simulink model "IonSatSimulation_ne_marche_pas_version_robin-lx-tavant.lab-lpp.local"  (R2019a)
settings: Solver=ode3  StartTime=0.0  StopTime=10000  FixedStep=.25  MaxStep=30  MinStep=.1  RelTol=1e-3
PreLoadFcn:
  | load('.\Data\SatConstants.mat')
model workspace (MAT data in the model file):
  repartition_matrix = Simulink.Parameter
  repartition_matrix.DataType = 'auto'
  repartition_matrix.Dimensions = [0 0]
  wheel_number = Simulink.Parameter
  wheel_number.Value = 3
  wheel_number.DataType = 'auto'
  wheel_number.Dimensions = [1 1]
undefined symbols (not defined in the file): Angle, Axis, deg, DiscIntNeverNeededParam, IAU, km, m, mu_Earth, rad, s, sat, X, Y, Z
libraries: aerolibutil x29, sm_lib x19, nesl_utility x16, aerolibconvert2 x13, vrlib x10, simulink x9, dspmathops x8, sharedtransform x7, sharedutil x5, aerolibgravity2 x4, sharedTrackingLibrary x2, aerolibcelestial x2
(part 1 of 3)
settings Model: SnapshotBufferSize=100  OrderedModelArguments=off  Creator=robin  LastModifiedBy=robin
settings SolverCC: InitialStep=.5  MaxConsecutiveMinStep=2
settings DataIOCC: SaveFormat=StructureWithTime  SaveOutput=off  SignalLogging=off  DSMLogging=off  SaveTime=off
settings OptimizationCC: DefaultParameterBehavior=Inlined  UseDivisionForNetSlopeComputation=on  GainParamInheritBuiltInType=on  UseFloatMulNetSlope=on  InlineInvariantSignals=on  PassReuseOutputArgsAs=Individual arguments  ZeroExternalMemoryAtStartup=off  ZeroInternalMemoryAtStartup=off  NoFixptDivByZeroProtection=on  EfficientFloat2IntCast=on  LifeSpan=1  OptimizeBlockOrder=speed  DifferentSizesBufferReuse=on
settings DebuggingCC: ParameterTunabilityLossMsg=error
settings HardwareCC: ProdBitPerInt=16  ProdBitPerPointer=8  ProdBitPerSizeT=24  ProdBitPerPtrDiffT=24  ProdLargestAtomicFloat=None  ProdWordSize=8  ProdLongLongMode=on  ProdHWDeviceType=Microchip->PIC18
settings SFSimCC: MATLABDynamicMemAlloc=off
settings RTWCC: SystemTargetFile=ert.tlc  TemplateMakefile=ert_default_tmf  GenerateReport=on  IncludeHyperlinkInReport=on  LaunchReport=on  GenerateTraceInfo=on  GenerateTraceReport=on  GenerateTraceReportSl=on  GenerateTraceReportSf=on  GenerateTraceReportEml=on  GenerateCodeMetricsReport=on
settings CodeAppCC: ForceParamTrailComments=on  IgnoreCustomStorageClasses=off  OperatorAnnotations=on  SimulinkDataObjDesc=on  SFDataObjDesc=on  CustomSymbolStrGlobalVar=rt$N$M  CustomSymbolStrType=$N$M  CustomSymbolStrFcn=$N$M$F  CustomSymbolStrMacro=$N$M  InsertBlockDesc=on
settings ERTTargetCC: TargetLangStandard=C99 (ISO)  GenerateSampleERTMain=on  IncludeMdlTerminateFcn=off  CombineSignalStateStructs=on  SupportAbsoluteTime=off  SupportComplex=off  SupportContinuousTime=on  SupportNonInlinedSFcns=on  InlinedParameterPlacement=NonHierarchical  ERTCustomFileTemplate=example_file_process.tlc  ERTFilePackagingFormat=CompactWithDataFile

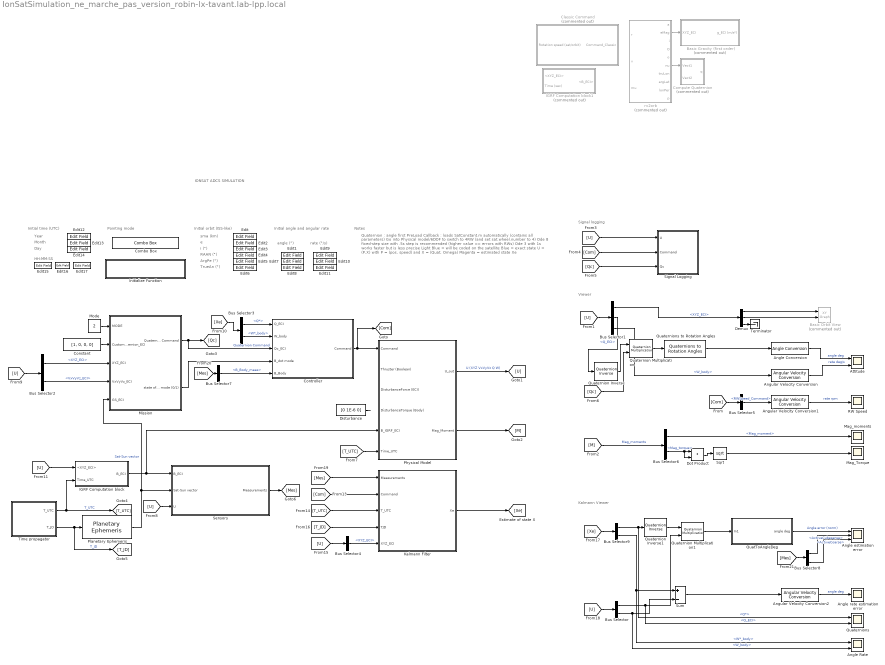
== system IonSatSimulation_ne_marche_pas_version_robin-lx-tavant.lab-lpp.local ==
  note: Kalmann Viewer
  note: IONSAT ADCS SIMULATION
  note: Viewer
  note: Pointing mode
  note: Initial orbit (ISS-like)
  note: sma (km)
  note: e
  note: i (°)
  note: RAAN (°)
  note: ArgPe (°)
  note: TrueAn (°)
  note: Initial angle and angular rate
  note: angle (°)
  note: rate (°/s)
  note: Notes
  note: Quaternion : angle first
      | PreLoad Callback : loads SatConstant.m automatically (contains all parameters)
      | Go into Physical model/6DOF to switch to 4RW (and set sat.wheel.number to 4)
      | Ode 8 fixed-step size with .5s step is recommended (higher value => errors with RWs)
      | Ode 3 with 1s works faster but is less precise
      | Light Blue = will be coded on the satellite
      | Blue = exact state U = (P,X) with P = (pos, speed) and X = (Quat, Omega)
      | Magenta = estimated state Xe
  note: Signal logging
  note: Month
  note: Year
  note: Day
  note: Initial time (UTC)
  note: HH:MM:SS
  Angle Conversion : aerolibconvert2/Angle Conversion  IU=rad  OU=deg
  Angle Rate : Scope  NumInputPorts=2
  Angle estimation error : Scope  NumInputPorts=3
  Angle rate estimation error : Scope
  Angular Velocity Conversion : aerolibconvert2/Angular Velocity Conversion  IU=rad/s  OU=deg/s
      settings: SourceProductName=Aerospace Blockset
  Angular Velocity Conversion1 : aerolibconvert2/Angular Velocity Conversion  IU=rad/s  OU=rpm
      settings: SourceProductName=Aerospace Blockset
  Angular Velocity Conversion2 : aerolibconvert2/Angular Velocity Conversion  IU=rad/s  OU=deg/s
      settings: SourceProductName=Aerospace Blockset
  Attitude : Scope  NumInputPorts=2
  Basic Gravity (first order) : Subsystem  Commented=on
  Basic Orbit View : simulink/Sinks/XY Graph  Commented=on  xmin=-10000000  xmax=10000000  ymin=-10000000  ymax=10000000  st=-1
  Bus Selector : BusSelector  OutputSignals=Q_ECI,W_body
  Bus Selector1 : BusSelector  OutputSignals=XYZ_ECI,Q_ECI,W_body
  Bus Selector2 : BusSelector  OutputSignals=XYZ_ECI,VxVyVz_ECI
  Bus Selector3 : BusSelector  OutputSignals=Q*,W*_body
  Bus Selector4 : BusSelector  OutputSignals=XYZ_ECI
  Bus Selector5 : BusSelector  OutputSignals=RWSpeed_Command
  Bus Selector6 : BusSelector  OutputSignals=Mag_moment,Mag_torque
  Bus Selector7 : BusSelector  OutputSignals=B_Body_meas
  Bus Selector8 : BusSelector  OutputSignals=ActiveCubesense,ActiveCoarse
  Bus Selector9 : BusSelector  OutputSignals=Q*,W*_body
  Classic Command : Subsystem  Commented=on
  Combo Box : ComboBox  LabelPosition=Hide  SelectedLabel=Sun Aero
      settings: Values={{'Nadir', 'Retrograde', 'Drag', 'Sun', 'Sun Aero', 'B-dot', 'Custom Quaternion'}, [1 5 4 3 2 6 7]}
  Compute Quaternion : Subsystem  Commented=on
  Constant : Constant  Value=[1, 0, 0, 0]
  Controller : Subsystem  TreatAsAtomicUnit=on
  Demux : Demux  Outputs=3
  Disturbance : Constant  Value=[0 1E-6 0]
  Dot Product : DotProduct  InputSameDT=on  OutDataTypeStr=Inherit: Inherit via internal rule
  Edit{,1..17} (18 alike) : EditField  LabelPosition=Hide  ShowInitialText=on  Alignment=Center
  IGRF Computation block : Subsystem
  IGRF Computation block1 : Subsystem  Commented=on
  Initialize Function : Subsystem  TreatAsAtomicUnit=on
  Kalmann Filter : Subsystem  TreatAsAtomicUnit=on  SystemSampleTime=1
  Mag_Torque : Scope
  Mag_moments : Scope
  Mission : Subsystem  TreatAsAtomicUnit=on  SystemSampleTime=1
  Mode : Constant  Value=2  OutDataTypeStr=int8
  Physical Model : Subsystem
      settings: MinAlgLoopOccurrences=on
  Planetary Ephemeris : aerolibcelestial/Planetary Ephemeris  kmflag=km,km/s  epochflag=Julian date  de=DE405  nCenter=Earth  nTarget=Sun  errorflag=Error  velflag=off
      settings: SourceProductName=Aerospace Blockset  SourceProductBaseCode=AE
  QuatToAngleDeg : Subsystem
  Quaternion Inverse : aerolibutil/Quaternion Inverse
      settings: SourceProductName=Aerospace Blockset
  Quaternion Inverse1 : aerolibutil/Quaternion Inverse
      settings: SourceProductName=Aerospace Blockset
  Quaternion Multiplication : aerolibutil/Quaternion Multiplication
  Quaternion Multiplication1 : aerolibutil/Quaternion Multiplication
  Quaternions : Scope  NumInputPorts=2
  Quaternions to Rotation Angles : sharedtransform/Quaternions to Rotation Angles  rotationOrder=ZYX  aMode=aMode
      settings: SourceProductBaseCode=AE
  RW Speed : Scope
  Sensors : Subsystem
  Signal Logging : Subsystem
  Sqrt : Sqrt  SaturateOnIntegerOverflow=on
  Sum : Sum  Inputs=+-
  Terminator : Terminator
  Time propagator : Subsystem
  rv2orb : MATLAB Function  Commented=on  TreatAsAtomicUnit=on
  wires:
  Mission/1(Quaternion Command) -> [Qc], Controller/3(Qc_ECI)  "Quaternion Command"
  Mode/1 -> Mission/1(MODE)
  Bus Selector2/2 -> Mission/4(VxVyVz_ECI)  "<VxVyVz_ECI>"
  Physical Model/1(U_out) -> [U]  "U (XYZ VxVyVz Q W)"
  Controller/1(Command) -> [Com], Physical Model/1(Command)
  Angle Conversion/1 -> Attitude/1  "angle deg"
  Demux/3 -> Terminator/1
  Demux/2 -> Basic Orbit View/2
  Angular Velocity Conversion/1 -> Attitude/2  "rate deg/s"
  Bus Selector1/1 -> Demux/1  "<XYZ_ECI>"
  Quaternion Multiplication/1 -> Quaternions to Rotation Angles/1
  Demux/1 -> Basic Orbit View/1
  Bus Selector1/3 -> Angular Velocity Conversion/1  "<W_body>"
  Quaternions to Rotation Angles/1 -> Angle Conversion/1
  Angular Velocity Conversion1/1 -> RW Speed/1  "rate rpm"
  [Com] -> Bus Selector5/1
  [U] -> Bus Selector1/1
  rv2orb/2(eMag) -> Basic Gravity (first order)/1(XYZ_ECI)
  Bus Selector2/1 -> Mission/3(XYZ_ECI)  "<XYZ_ECI>"
  rv2orb/6(nu) -> Compute Quaternion/1(Vect1)
  Bus Selector3/1 -> Controller/1(Q_ECI)  "<Q*>"
  Bus Selector3/2 -> Controller/2(W_body)  "<W*_body>"
  Planetary Ephemeris/1 -> Mission/5(GS_ECI), Sensors/2(Sat-Sun vector)  "Sat-Sun vector"
  [U] -> Signal Logging/1(U)
  [Com] -> Signal Logging/2(Command)
  [Qc] -> Signal Logging/3(Qc)
  [Qc] -> Quaternion Multiplication/2
  Quaternion Inverse/1 -> Quaternion Multiplication/1
  Bus Selector1/2 -> Quaternion Inverse/1  "<Q_ECI>"
  Physical Model/2(Mag_Moment) -> [M]
  [M] -> Bus Selector6/1  "Mag_moments"
  Time propagator/1(T_UTC) -> [T_UTC], IGRF Computation block/2("Time_UTC ")  "T_UTC"
  Time propagator/2(T_JD) -> [T_JD], Planetary Ephemeris/1  "T_JD"
  Disturbance/1 -> ?
  Mission/2(state of B-dot mode (0/1)) -> Controller/4(B_dot mode)
  IGRF Computation block/1(B_ECI) -> Physical Model/5(B_IGRF_ECI), Sensors/1(B_ECI)
  Constant/1 -> Mission/2(Custom Quaternion_ECI)
  [T_UTC] -> Physical Model/6(Time_UTC)
  [U] -> Bus Selector2/1
  [Xe] -> Bus Selector3/1
  [U] -> IGRF Computation block/1(<XYZ_ECI>)
  Kalmann Filter/1(Xe) -> [Xe]
  [Com] -> Kalmann Filter/2(Command)
  [T_UTC] -> Kalmann Filter/3(T_UTC)
  [U] -> Bus Selector4/1
  Bus Selector4/1 -> Kalmann Filter/5(XYZ_ECI)  "<XYZ_ECI>"
  [T_JD] -> Kalmann Filter/4(TJD)
  [Xe] -> Bus Selector9/1
  [U] -> Bus Selector/1
  Bus Selector9/2 -> Angle Rate/1, Sum/1  "<W*_body>"
  Bus Selector/2 -> Angle Rate/2, Sum/2  "<W_body>"
  Sum/1 -> Angular Velocity Conversion2/1
  Bus Selector9/1 -> Quaternions/1, Quaternion Inverse1/1  "<Q*>"
  Quaternion Inverse1/1 -> Quaternion Multiplication1/1
  Bus Selector/1 -> Quaternions/2, Quaternion Multiplication1/2  "<Q_ECI>"
  Angular Velocity Conversion2/1 -> Angle rate estimation error/1  "angle deg"
  Bus Selector5/1 -> Angular Velocity Conversion1/1  "<RWSpeed_Command>"
  Bus Selector6/1 -> Mag_moments/1  "<Mag_moment>"
  Bus Selector6/2 -> Dot Product/2, Dot Product/1  "<Mag_torque>"
  Dot Product/1 -> Sqrt/1
  Sqrt/1 -> Mag_Torque/1
  Bus Selector7/1 -> Controller/5(B_Body)  "<B_Body_meas>"
  [U] -> Sensors/3(U)
  Sensors/1(Measurements) -> [Mes]
  [Mes] -> Kalmann Filter/1(Measurements)
  [Mes] -> Bus Selector7/1
  [Mes] -> Bus Selector8/1
  Bus Selector8/1 -> Angle estimation error/2  "<ActiveCubesense>"
  Bus Selector8/2 -> Angle estimation error/3  "<ActiveCoarse>"
  Quaternion Multiplication1/1 -> QuatToAngleDeg/1(In1)
  QuatToAngleDeg/1(angle deg) -> Angle estimation error/1  "Angle error (norm)"

== system IonSatSimulation_ne_marche_pas_version_robin-lx-tavant.lab-lpp.local/Basic Gravity (first order) ==
  XYZ_ECI : Inport
  Constant : Constant  Value=-mu_Earth
  Constant3 : Constant  Value=3/2
  Divide : Product  Inputs=*/
  Norm : Subsystem
  Product : Product
  Square3 : Math  Operator=pow  SaturateOnIntegerOverflow=on
  g_ECI (m/s²) : Outport  VectorParamsAs1DForOutWhenUnconnected=on
  wires:
  Constant/1 -> Divide/1
  Divide/1 -> Product/2
  Product/1 -> g_ECI (m/s²)/1
  XYZ_ECI/1 -> Norm/1(u), Product/1
  Square3/1 -> Divide/2  "r**3"
  Constant3/1 -> Square3/2
  Norm/1(r**2) -> Square3/1

== system IonSatSimulation_ne_marche_pas_version_robin-lx-tavant.lab-lpp.local/Classic Command ==
  Rotation speed (sat/orbit) : Inport
  Gain : Gain  Gain=- sat.PID.k_mag_classic
  Command_Classic : Outport
  wires:
  Rotation speed (sat/orbit)/1 -> Gain/1
  Gain/1 -> Command_Classic/1

== system IonSatSimulation_ne_marche_pas_version_robin-lx-tavant.lab-lpp.local/Compute Quaternion ==
  Vect1 : Inport
  Vect2 : Inport  Port=2
  Constant : Constant
  Cross Product : vrlib/Utilities/Cross Product
      settings: SourceProductName=Simulink
  Dot Product : DotProduct  InputSameDT=on  OutDataTypeStr=Inherit: Inherit via internal rule
  Mux : Mux  Inputs=2
  Normalization : dspmathops/Normalization  NormType=2-norm  Bias=1e-10  NormOver=Each column  Dimension=1  roundingMode=Floor  overflowMode=off  accumDataTypeStr=Inherit: Same as product output  accumLastDataTypeStr=Inherit: Same as product output  outputDataTypeStr=Inherit: Same as product output  outputMin=[]  outputMax=[]  outputLastDataTypeStr=Inherit: Same as product output
      settings: SourceProductName=DSP System Toolbox
  Normalization1 : dspmathops/Normalization  NormType=2-norm  Bias=1e-10  NormOver=Each column  Dimension=1  roundingMode=Floor  overflowMode=off  accumDataTypeStr=Inherit: Same as product output  accumLastDataTypeStr=Inherit: Same as product output  outputDataTypeStr=Inherit: Same as product output  outputMin=[]  outputMax=[]  outputLastDataTypeStr=Inherit: Same as product output
      settings: SourceProductName=DSP System Toolbox
  Quaternion Normalize : sharedutil/Quaternion Normalize  aMode=aMode
      settings: SourceProductName=Aerospace Blockset  SourceProductBaseCode=AE
  Sum : Sum  Inputs=|++
  q : Outport  PortDimensions=4
  wires:
  Vect1/1 -> Normalization/1
  Normalization/1 -> Cross Product/1, Dot Product/1
  Vect2/1 -> Normalization1/1
  Normalization1/1 -> Dot Product/2, Cross Product/2
  Cross Product/1 -> Mux/2
  Dot Product/1 -> Sum/1
  Sum/1 -> Mux/1
  Constant/1 -> Sum/2
  Mux/1 -> Quaternion Normalize/1
  Quaternion Normalize/1 -> q/1

== system IonSatSimulation_ne_marche_pas_version_robin-lx-tavant.lab-lpp.local/Controller ==
  note: Choix d'un contrôleur PID : plus simple et robuste qu'un LQR/SliddingSurface ou autre
  note: Runs as fast as possible
  note: Runs at 1Hz
  Q_ECI : Inport
  W_body : Inport  Port=2
  Qc_ECI : Inport  Port=3
  B_dot mode : Inport  Port=4
  B_Body : Inport  Port=5
  B-dot choice1 : Subsystem
  B-dot choice2 : Subsystem
  B-dot command : Subsystem  TreatAsAtomicUnit=on
  Bus Creator : BusCreator  Inputs=2
  Ground2 : Ground  Commented=on
  PID (nominal command) : Subsystem  TreatAsAtomicUnit=on  SystemSampleTime=1
  RW4 : Subsystem  Commented=on
  Command : Outport
  wires:
  Ground2/1 -> RW4/1(Mc (scalar))
  B_Body/1 -> B-dot command/1(B), PID (nominal command)/4(B_IGRF_Body)
  B-dot choice2/1(output command) -> Bus Creator/2  "Magnetotorquer_Command"
  B-dot choice1/1(output command) -> Bus Creator/1  "RWSpeed_Command"
  B-dot command/2(Wheel command (0)) -> B-dot choice1/2(Command (B-dot))
  B-dot command/1(Magnetic moment (B-dot)) -> B-dot choice2/2(Command (B-dot))
  B_dot mode/1 -> B-dot choice2/3(B_dot mode (0/1)), B-dot choice1/3(B_dot mode (0/1))
  Q_ECI/1 -> PID (nominal command)/1(Q_ECI)
  Qc_ECI/1 -> PID (nominal command)/2(Qc_ECI)
  W_body/1 -> PID (nominal command)/3(W_Body)
  PID (nominal command)/1(RW Command) -> B-dot choice1/1(" command (normal)")
  PID (nominal command)/2(Mag Command) -> B-dot choice2/1(" command (normal)")
  Bus Creator/1 -> Command/1

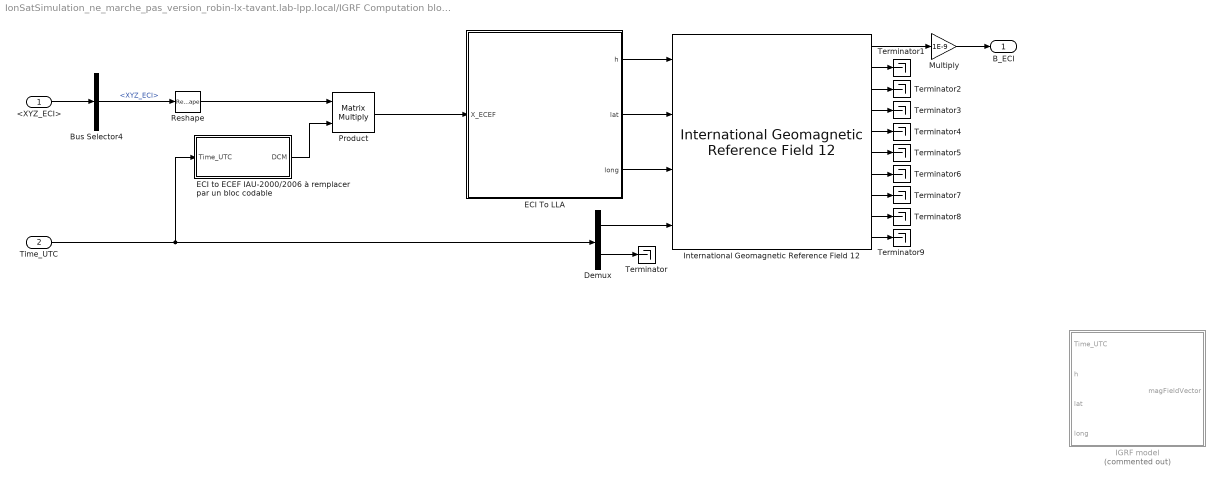
== system IonSatSimulation_ne_marche_pas_version_robin-lx-tavant.lab-lpp.local/IGRF Computation block ==
  <XYZ_ECI> : Inport
  "Time_UTC " : Inport  Port=2
  Bus Selector4 : BusSelector  OutputSignals=XYZ_ECI
  Demux : Demux  Outputs=2
  ECI To LLA : MATLAB Function  TreatAsAtomicUnit=on
  ECI to ECEF IAU-2000/2006 à remplacer par un bloc codable : MATLAB Function  TreatAsAtomicUnit=on
  IGRF model : MATLAB Function  Commented=on  TreatAsAtomicUnit=on
  International Geomagnetic Reference Field 12 : aerolibgravity2/International Geomagnetic Reference Field 12  units=Metric (MKS)  time_in=on  month=January  day=1  year=2020  action=None  sv_out=on
      settings: SourceProductName=Aerospace Blockset  SourceProductBaseCode=AE
  Multiply : Gain  Gain=1E-9
  Product : Product  Multiplication=Matrix(*)
  Reshape : Reshape  OutputDimensionality=Row vector (2-D)
  Terminator{,1..9} (10 alike) : Terminator
  B_ECI : Outport
  wires:
  ECI To LLA/3(long) -> International Geomagnetic Reference Field 12/3
  ECI To LLA/2(lat) -> International Geomagnetic Reference Field 12/2
  ECI To LLA/1(h) -> International Geomagnetic Reference Field 12/1
  International Geomagnetic Reference Field 12/1 -> Multiply/1
  Demux/1 -> International Geomagnetic Reference Field 12/4
  Demux/2 -> Terminator/1
  International Geomagnetic Reference Field 12/2 -> Terminator1/1
  International Geomagnetic Reference Field 12/3 -> Terminator2/1
  International Geomagnetic Reference Field 12/4 -> Terminator3/1
  International Geomagnetic Reference Field 12/5 -> Terminator4/1
  International Geomagnetic Reference Field 12/6 -> Terminator5/1
  International Geomagnetic Reference Field 12/7 -> Terminator6/1
  International Geomagnetic Reference Field 12/8 -> Terminator7/1
  International Geomagnetic Reference Field 12/9 -> Terminator8/1
  International Geomagnetic Reference Field 12/10 -> Terminator9/1
  Multiply/1 -> B_ECI/1
  ECI to ECEF IAU-2000/2006 à remplacer par un bloc codable/1(DCM) -> Product/2
  "Time_UTC "/1 -> Demux/1, ECI to ECEF IAU-2000/2006 à remplacer par un bloc codable/1(Time_UTC)
  <XYZ_ECI>/1 -> Bus Selector4/1
  Reshape/1 -> Product/1
  Product/1 -> ECI To LLA/1(X_ECEF)
  Bus Selector4/1 -> Reshape/1  "<XYZ_ECI>"

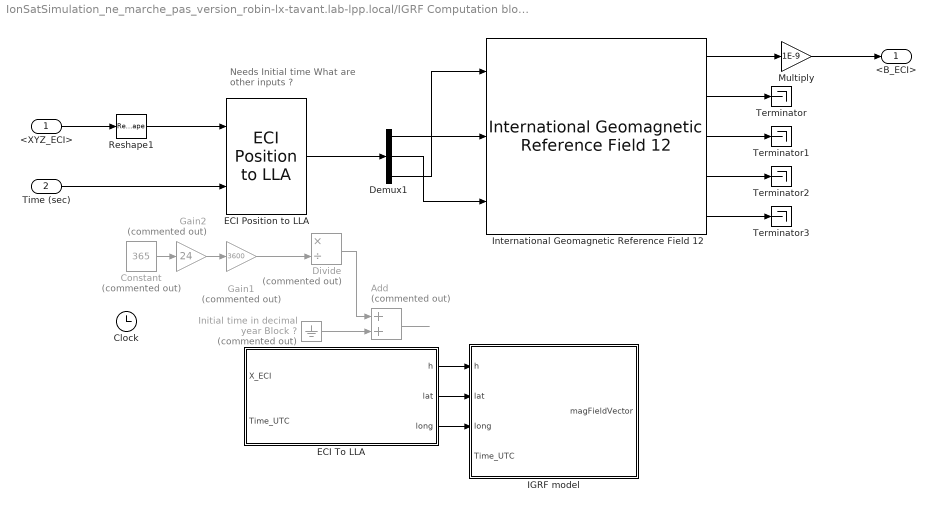
== system IonSatSimulation_ne_marche_pas_version_robin-lx-tavant.lab-lpp.local/IGRF Computation block1 ==
  note: Needs Initial time
      | What are other inputs ?
  <XYZ_ECI> : Inport
  Time (sec) : Inport  Port=2
  Add : Sum  Commented=on
  Clock : Clock
  Constant : Constant  Commented=on  Value=365
  Demux1 : Demux  Outputs=3
  Divide : Product  Commented=on  Inputs=*/
  ECI Position to LLA : aerolibtransform2/ECI Position to LLA  red=IAU-2000/2006  year=2020  month=January  day=1  hour=0  min=0  sec=0  deltaT=Sec  errorflag=Error  extraparamflag=off  eunits=Metric (MKS)  earthmodel=WGS84  flat=1/298.257223563  eqradius=6378137
      settings: AttributesFormatString=%<red>  SourceProductName=Aerospace Blockset  SourceProductBaseCode=AE
  ECI To LLA : MATLAB Function  TreatAsAtomicUnit=on
  Gain1 : Gain  Commented=on  Gain=3600
  Gain2 : Gain  Commented=on  Gain=24
  IGRF model : MATLAB Function  TreatAsAtomicUnit=on
  Initial time in decimal year Block ? : Ground  Commented=on
  International Geomagnetic Reference Field 12 : aerolibgravity2/International Geomagnetic Reference Field 12  units=Metric (MKS)  time_in=off  month=January  day=1  year=2020  action=None  sv_out=off
      settings: SourceProductName=Aerospace Blockset  SourceProductBaseCode=AE
  Multiply : Gain  Gain=1E-9
  Reshape1 : Reshape  OutputDimensionality=Column vector (2-D)
  Terminator{,1..3} (4 alike) : Terminator
  <B_ECI> : Outport
  wires:
  International Geomagnetic Reference Field 12/1 -> Multiply/1
  Demux1/2 -> International Geomagnetic Reference Field 12/3
  Time (sec)/1 -> ECI Position to LLA/2
  ECI Position to LLA/1 -> Demux1/1
  <XYZ_ECI>/1 -> Reshape1/1
  Gain2/1 -> Gain1/1
  Constant/1 -> Gain2/1
  Gain1/1 -> Divide/2
  Add/1 -> ?
  Divide/1 -> Add/1
  Initial time in decimal year Block ?/1 -> Add/2
  Reshape1/1 -> ECI Position to LLA/1
  International Geomagnetic Reference Field 12/3 -> Terminator1/1
  International Geomagnetic Reference Field 12/2 -> Terminator/1
  International Geomagnetic Reference Field 12/4 -> Terminator2/1
  International Geomagnetic Reference Field 12/5 -> Terminator3/1
  Demux1/1 -> International Geomagnetic Reference Field 12/2
  Demux1/3 -> International Geomagnetic Reference Field 12/1
  Multiply/1 -> <B_ECI>/1
  ECI To LLA/3(long) -> IGRF model/3(long)
  ECI To LLA/2(lat) -> IGRF model/2(lat)
  ECI To LLA/1(h) -> IGRF model/1(h)

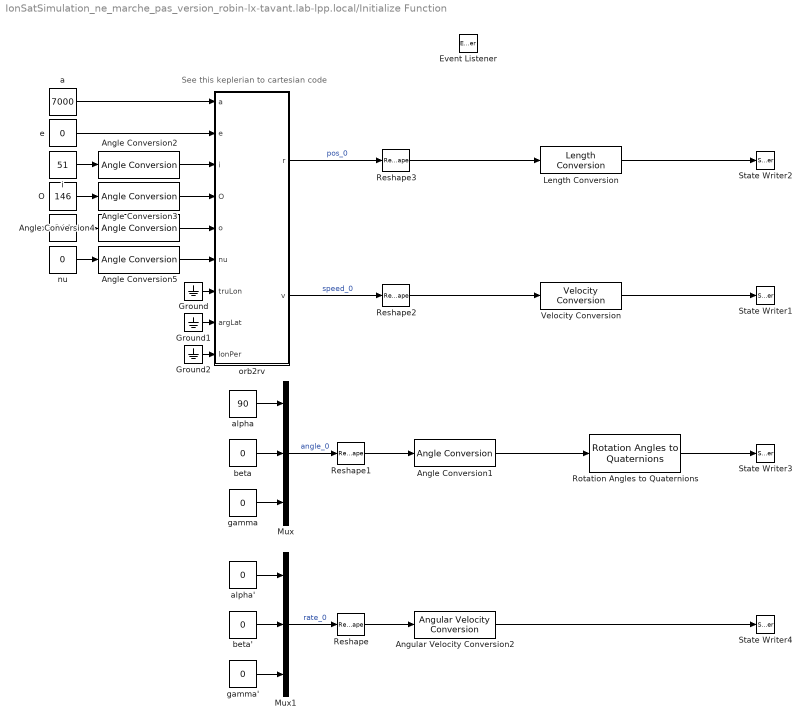
== system IonSatSimulation_ne_marche_pas_version_robin-lx-tavant.lab-lpp.local/Initialize Function ==
  note: See this keplerian to cartesian code
  Angle Conversion{1..5} (5 alike) : aerolibconvert2/Angle Conversion  IU=deg  OU=rad
  Angular Velocity Conversion2 : aerolibconvert2/Angular Velocity Conversion  IU=deg/s  OU=rad/s
      settings: SourceProductName=Aerospace Blockset
  Event Listener : EventListener  DisableCoverage=on  EventName=reset
  Ground : Ground
  Ground1 : Ground
  Ground2 : Ground
  Length Conversion : aerolibconvert2/Length Conversion  IU=km  OU=m
  Mux : Mux  Inputs=3
  Mux1 : Mux  Inputs=3
  O : Constant  Value=146
  Reshape{,1..3} (4 alike) : Reshape  OutputDimensionality=Column vector (2-D)
  Rotation Angles to Quaternions : sharedtransform/Rotation Angles to Quaternions  rotationOrder=ZYX  aMode=aMode
      settings: SourceProductName=Aerospace Blockset  SourceProductBaseCode=AE
  State Writer1 : StateWriter  StateOwnerBlock=../../Physical Model/6DOF in ECI frame/Integrator_speed
  State Writer2 : StateWriter  StateOwnerBlock=../../Physical Model/6DOF in ECI frame/Integrator_pos
  State Writer3 : StateWriter  StateOwnerBlock=../../Physical Model/6DOF in ECI frame/Compute Q_ECI/Integrator_quat
  State Writer4 : StateWriter  StateOwnerBlock=../../Physical Model/6DOF in ECI frame/Integrator_rate
  Velocity Conversion : aerolibconvert2/Velocity Conversion  IU=km/s  OU=m/s
  a : Constant  Value=7000
  alpha : Constant  Value=90
  alpha' : Constant  Value=0
  beta : Constant  Value=0
  beta' : Constant  Value=0
  e : Constant  Value=0
  gamma : Constant  Value=0
  gamma' : Constant  Value=0
  i : Constant  Value=51
  nu : Constant  Value=0
  o : Constant  Value=344
  orb2rv : MATLAB Function  TreatAsAtomicUnit=on
  wires:
  Angular Velocity Conversion2/1 -> State Writer4/1
  Angle Conversion1/1 -> Rotation Angles to Quaternions/1
  orb2rv/1(r) -> Reshape3/1  "pos_0"
  Mux1/1 -> Reshape/1  "rate_0"
  Mux/1 -> Reshape1/1  "angle_0"
  orb2rv/2(v) -> Reshape2/1  "speed_0"
  Rotation Angles to Quaternions/1 -> State Writer3/1
  Reshape/1 -> Angular Velocity Conversion2/1
  Reshape1/1 -> Angle Conversion1/1
  Reshape2/1 -> Velocity Conversion/1
  Reshape3/1 -> Length Conversion/1
  a/1 -> orb2rv/1(a)
  e/1 -> orb2rv/2(e)
  i/1 -> Angle Conversion2/1
  O/1 -> Angle Conversion3/1
  o/1 -> Angle Conversion4/1
  nu/1 -> Angle Conversion5/1
  Angle Conversion2/1 -> orb2rv/3(i)
  Angle Conversion3/1 -> orb2rv/4(O)
  Angle Conversion4/1 -> orb2rv/5(o)
  Angle Conversion5/1 -> orb2rv/6(nu)
  Ground/1 -> orb2rv/7(truLon)
  Ground1/1 -> orb2rv/8(argLat)
  Ground2/1 -> orb2rv/9(lonPer)
  Length Conversion/1 -> State Writer2/1
  Velocity Conversion/1 -> State Writer1/1
  alpha/1 -> Mux/1
  beta/1 -> Mux/2
  gamma/1 -> Mux/3
  alpha'/1 -> Mux1/1
  gamma'/1 -> Mux1/3
  beta'/1 -> Mux1/2

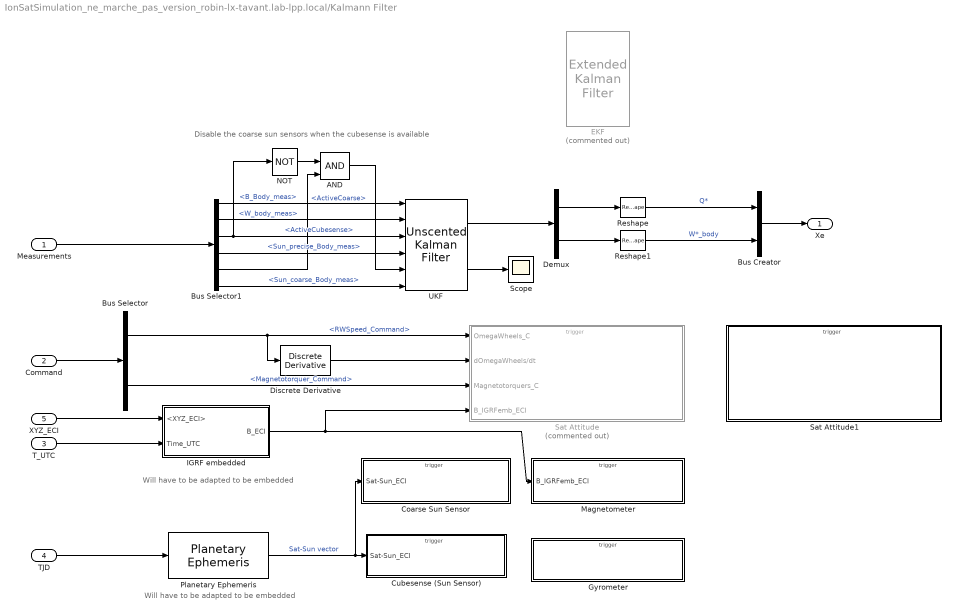
== system IonSatSimulation_ne_marche_pas_version_robin-lx-tavant.lab-lpp.local/Kalmann Filter ==
  note: Disable the coarse sun sensors when the cubesense is available
  note: Will have to be adapted to be embedded
  note: Will have to be adapted to be embedded
  Measurements : Inport
  Command : Inport  Port=2
  T_UTC : Inport  Port=3
  TJD : Inport  Port=4
  XYZ_ECI : Inport  Port=5
  AND : Logic  IconShape=distinctive  AllPortsSameDT=off  OutDataTypeStr=boolean
  Bus Creator : BusCreator  Inputs=2
  Bus Selector : BusSelector  OutputSignals=RWSpeed_Command,Magnetotorquer_Command
  Bus Selector1 : BusSelector  OutputSignals=B_Body_meas,W_body_meas,ActiveCubesense,Sun_precise_Body_meas,ActiveCoarse,Sun_coarse_Body_meas
  Coarse Sun Sensor : Subsystem  TreatAsAtomicUnit=on
  Cubesense (Sun Sensor) : Subsystem  TreatAsAtomicUnit=on
  Demux : Demux  Outputs=2
  Discrete Derivative : simulink/Discrete/Discrete Derivative  gainval=1.0  ICPrevScaledInput=0.0  OutMin=[]  OutMax=[]  OutDataType=fixdt(1, 16)  OutScaling=2^-10  DoSatur=off
  EKF : sharedTrackingLibrary/Extended Kalman Filter  Commented=on  StateTransitionFcn=SatAttitude  HasStateTransitionJacobianFcn=off  HasAdditiveProcessNoise=Additive  ProcessNoise=1e-10  HasTimeVaryingProcessNoise=off  HasStateTransitionFcnExtraArgument=0  InitialState=[1 0 0 0 0 0 0]  InitialStateCovariance=1  MeasurementFcn1=MagMeasure  HasMeasurementJacobianFcn1=off  HasMeasurementEnablePort1=off  HasAdditiveMeasurementNoise1=Additive  MeasurementNoise1=sat.sensors.mag_sigma*sat.sensors.mag_sigma*ones(3,1)  HasTimeVaryingMeasurementNoise1=off  HasMeasurementFcnExtraArgument1=0  MeasurementFcn2=GyroMeasure  HasMeasurementJacobianFcn2=off  HasMeasurementEnablePort2=off  HasAdditiveMeasurementNoise2=Additive  MeasurementNoise2=sat.sensors.gyro_sigma*sat.sensors.gyro_sigma*ones(3,1)  HasTimeVaryingMeasurementNoise2=off  HasMeasurementFcnExtraArgument2=0  MeasurementFcn3=SunMeasure  HasMeasurementJacobianFcn3=off  HasMeasurementEnablePort3=on  HasAdditiveMeasurementNoise3=Additive  MeasurementNoise3=sat.sensors.sun_sigma*sat.sensors.sun_sigma*ones(3,1)  HasTimeVaryingMeasurementNoise3=off  HasMeasurementFcnExtraArgument3=0  MeasurementFcn4=SunMeasureCoarse  HasMeasurementJacobianFcn4=off  HasMeasurementEnablePort4=on  HasAdditiveMeasurementNoise4=Additive  MeasurementNoise4=sat.sensors.sun_coarse_sigma*sat.sensors.sun_coarse_sigma*ones(3,1)  HasTimeVaryingMeasurementNoise4=off  HasMeasurementFcnExtraArgument4=0  MeasurementFcn5=myMeasurementFcn  HasMeasurementJacobianFcn5=off  HasMeasurementEnablePort5=off  HasAdditiveMeasurementNoise5=Additive  MeasurementNoise5=1  HasTimeVaryingMeasurementNoise5=off  HasMeasurementFcnExtraArgument5=0  EnableMultirate=off  StateTransitionFcnSampleTime=1  MeasurementFcn1SampleTime=1  MeasurementFcn2SampleTime=1  MeasurementFcn3SampleTime=1  MeasurementFcn4SampleTime=1  MeasurementFcn5SampleTime=1  UseCurrentEstimator=on  OutputStateCovariance=off  DataType=double  SampleTime=1  NumberOfMeasurements=4
      settings: SourceProductName=Control System Toolbox  SourceProductBaseCode=CT
  Gyrometer : Subsystem  TreatAsAtomicUnit=on
  IGRF embedded : Subsystem
  Magnetometer : Subsystem  TreatAsAtomicUnit=on
  NOT : Logic  Operator=NOT  IconShape=distinctive  AllPortsSameDT=off  OutDataTypeStr=boolean
  Planetary Ephemeris : aerolibcelestial/Planetary Ephemeris  kmflag=km,km/s  epochflag=Julian date  de=DE405  nCenter=Earth  nTarget=Sun  errorflag=Error  velflag=off
      settings: SourceProductName=Aerospace Blockset  SourceProductBaseCode=AE
  Reshape : Reshape  OutputDimensionality=Customize  OutputDimensions=[4]
  Reshape1 : Reshape  OutputDimensionality=Customize  OutputDimensions=[3]
  Sat Attitude : Subsystem  Commented=on  TreatAsAtomicUnit=on
  Sat Attitude1 : Subsystem  TreatAsAtomicUnit=on
  Scope : Scope
  UKF : sharedTrackingLibrary/Unscented Kalman Filter  StateTransitionFcn=SatAttitude  HasAdditiveProcessNoise=Additive  ProcessNoise=5e-7  HasTimeVaryingProcessNoise=off  HasStateTransitionFcnExtraArgument=0  InitialState=[1 0 0 0 0 0 0]  InitialStateCovariance=1e-7  Alpha=3e-2  Beta=2  Kappa=0  MeasurementFcn1=MagMeasure  HasMeasurementEnablePort1=off  HasAdditiveMeasurementNoise1=Additive  MeasurementNoise1=sat.sensors.mag_sigma*sat.sensors.mag_sigma*ones(3,1)  HasTimeVaryingMeasurementNoise1=off  HasMeasurementFcnExtraArgument1=0  MeasurementFcn2=GyroMeasure  HasMeasurementEnablePort2=off  HasAdditiveMeasurementNoise2=Additive  MeasurementNoise2=sat.sensors.gyro_sigma*sat.sensors.gyro_sigma*ones(3,1)  HasTimeVaryingMeasurementNoise2=off  HasMeasurementFcnExtraArgument2=0  MeasurementFcn3=SunMeasure  HasMeasurementEnablePort3=on  HasAdditiveMeasurementNoise3=Additive  MeasurementNoise3=sat.sensors.sun_sigma*sat.sensors.sun_sigma*ones(3,1)  HasTimeVaryingMeasurementNoise3=off  HasMeasurementFcnExtraArgument3=0  MeasurementFcn4=SunMeasureCoarse  HasMeasurementEnablePort4=on  HasAdditiveMeasurementNoise4=Additive  MeasurementNoise4=sat.sensors.sun_coarse_sigma*sat.sensors.sun_coarse_sigma*ones(3,1)  HasTimeVaryingMeasurementNoise4=off  HasMeasurementFcnExtraArgument4=0  MeasurementFcn5=myMeasurementFcn  HasMeasurementEnablePort5=off  HasAdditiveMeasurementNoise5=Additive  MeasurementNoise5=1  HasTimeVaryingMeasurementNoise5=off  HasMeasurementFcnExtraArgument5=0  EnableMultirate=off  StateTransitionFcnSampleTime=1  MeasurementFcn1SampleTime=1  MeasurementFcn2SampleTime=1  MeasurementFcn3SampleTime=1  MeasurementFcn4SampleTime=1  MeasurementFcn5SampleTime=1  UseCurrentEstimator=on  OutputStateCovariance=on  DataType=double  SampleTime=1  NumberOfMeasurements=4
      settings: SourceProductName=Control System Toolbox  SourceProductBaseCode=CT
  Xe : Outport
  wires:
  Measurements/1 -> Bus Selector1/1
  UKF/1 -> Demux/1
  XYZ_ECI/1 -> IGRF embedded/1(<XYZ_ECI>)
  T_UTC/1 -> IGRF embedded/2("Time_UTC ")
  IGRF embedded/1(B_ECI) -> Sat Attitude/4(B_IGRFemb_ECI), Magnetometer/1(B_IGRFemb_ECI)
  Command/1 -> Bus Selector/1
  Bus Selector/1 -> Discrete Derivative/1, Sat Attitude/1(OmegaWheels_C)  "<RWSpeed_Command>"
  Bus Selector/2 -> Sat Attitude/3(Magnetotorquers_C)  "<Magnetotorquer_Command>"
  TJD/1 -> Planetary Ephemeris/1
  Bus Selector1/1 -> UKF/1  "<B_Body_meas>"
  Bus Selector1/2 -> UKF/2  "<W_body_meas>"
  Bus Selector1/6 -> UKF/6  "<Sun_coarse_Body_meas>"
  Planetary Ephemeris/1 -> Coarse Sun Sensor/1(Sat-Sun_ECI), Cubesense (Sun Sensor)/1(Sat-Sun_ECI)  "Sat-Sun vector"
  Discrete Derivative/1 -> Sat Attitude/2(dOmegaWheels/dt)
  Bus Selector1/3 -> UKF/3, NOT/1  "<ActiveCubesense>"
  Bus Selector1/4 -> UKF/4  "<Sun_precise_Body_meas>"
  Bus Selector1/5 -> AND/2  "<ActiveCoarse>"
  NOT/1 -> AND/1
  AND/1 -> UKF/5
  UKF/2 -> Scope/1
  Bus Creator/1 -> Xe/1
  Demux/1 -> Reshape/1
  Demux/2 -> Reshape1/1
  Reshape/1 -> Bus Creator/1  "Q*"
  Reshape1/1 -> Bus Creator/2  "W*_body"

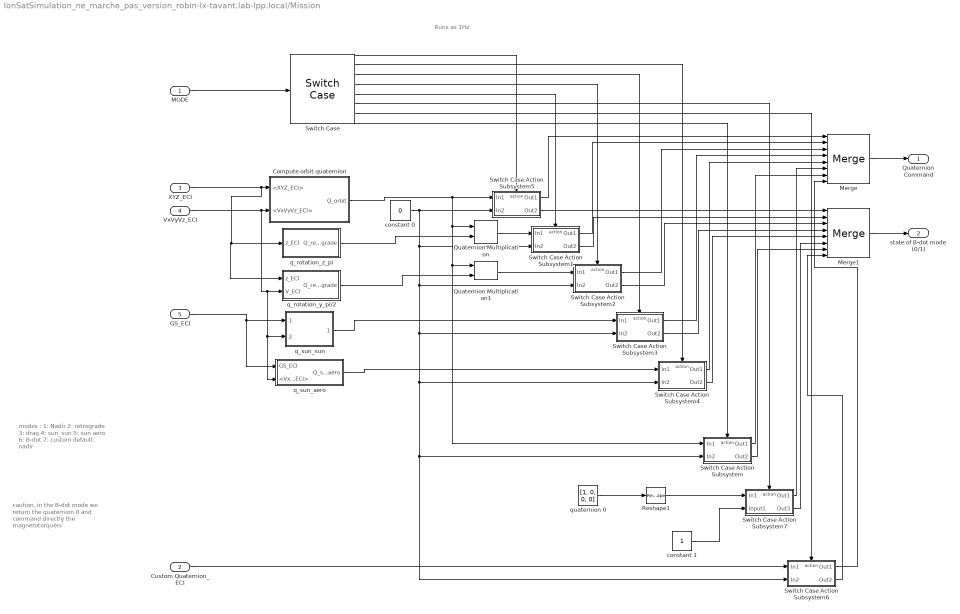
== system IonSatSimulation_ne_marche_pas_version_robin-lx-tavant.lab-lpp.local/Mission ==
  note: caution, in the B-dot mode we return the quaternion 0 and command directly the magnetotorquers
  note: modes :
      | 1: Nadir
      | 2: retrograde
      | 3: drag
      | 4: sun_sun
      | 5: sun aero
      | 6: B-dot
      | 7: custom
      | default: nadir
  note: Runs as 1Hz
  MODE : Inport  OutMin=1  OutMax=100  OutDataTypeStr=int8
  Custom Quaternion_ECI : Inport  Port=2
  XYZ_ECI : Inport  Port=3
  VxVyVz_ECI : Inport  Port=4
  GS_ECI : Inport  Port=5
  Compute orbit quaternion : Subsystem
  Merge : Merge  Inputs=8
  Merge1 : Merge  Inputs=8
  Quaternion Multiplication : aerolibutil/Quaternion Multiplication
  Quaternion Multiplication1 : aerolibutil/Quaternion Multiplication
  Reshape1 : Reshape  OutputDimensionality=Column vector (2-D)
  Switch Case : SwitchCase  CaseConditions={1, 2, 3, 4, 5, 6, 7}
  Switch Case Action Subsystem : Subsystem  TreatAsAtomicUnit=on
  Switch Case Action Subsystem1 : Subsystem  TreatAsAtomicUnit=on
  Switch Case Action Subsystem2 : Subsystem  TreatAsAtomicUnit=on
  Switch Case Action Subsystem3 : Subsystem  TreatAsAtomicUnit=on
  Switch Case Action Subsystem4 : Subsystem  TreatAsAtomicUnit=on
  Switch Case Action Subsystem5 : Subsystem  TreatAsAtomicUnit=on
  Switch Case Action Subsystem6 : Subsystem  TreatAsAtomicUnit=on
  Switch Case Action Subsystem7 : Subsystem  TreatAsAtomicUnit=on
  constant 0 : Constant  Value=0
  constant 1 : Constant
  q_rotation_y_pi/2 : Subsystem
  q_rotation_z_pi : Subsystem
  q_sun_aero : Subsystem
  q_sun_sun : Subsystem
  quaternion 0 : Constant  Value=[1, 0, 0, 0]
  Quaternion Command : Outport
  state of B-dot mode (0/1) : Outport  Port=2
  wires:
  q_sun_sun/1(Q_sun_sun) -> Switch Case Action Subsystem3/1(In1)
  GS_ECI/1 -> q_sun_aero/1(GS_ECI), q_sun_sun/1(<VxVyVz_ECI>)
  MODE/1 -> Switch Case/1
  q_rotation_y_pi/2/1(Q_retrograde) -> Quaternion Multiplication1/2
  Switch Case/3 -> Switch Case Action Subsystem3/Action
  q_sun_aero/1(Q_sun_aero) -> Switch Case Action Subsystem4/1(In1)
  Merge/1 -> Quaternion Command/1
  XYZ_ECI/1 -> q_rotation_z_pi/1(z_ECI), q_rotation_y_pi/2/1(z_ECI), Compute orbit quaternion/1(<XYZ_ECI>)
  Switch Case/5 -> Switch Case Action Subsystem1/Action
  q_rotation_z_pi/1(Q_retrograde) -> Quaternion Multiplication/2
  Switch Case/4 -> Switch Case Action Subsystem2/Action
  quaternion 0/1 -> Reshape1/1
  VxVyVz_ECI/1 -> q_sun_aero/2(<VxVyVz_ECI>), q_sun_sun/2(GS_ECI), q_rotation_y_pi/2/2(V_ECI), Compute orbit quaternion/2(<VxVyVz_ECI>)
  Switch Case/2 -> Switch Case Action Subsystem4/Action
  Quaternion Multiplication1/1 -> Switch Case Action Subsystem2/1(In1)
  Compute orbit quaternion/1(Q_orbit) -> Switch Case Action Subsystem/1(In1), Quaternion Multiplication1/1, Quaternion Multiplication/1, Switch Case Action Subsystem5/1(In1)
  Switch Case/6 -> Switch Case Action Subsystem7/Action
  Quaternion Multiplication/1 -> Switch Case Action Subsystem1/1(In1)
  Reshape1/1 -> Switch Case Action Subsystem7/1(In1)
  constant 0/1 -> Switch Case Action Subsystem6/2(In2), Switch Case Action Subsystem/2(In2), Switch Case Action Subsystem4/2(In2), Switch Case Action Subsystem3/2(In2), Switch Case Action Subsystem2/2(In2), Switch Case Action Subsystem1/2(In2), Switch Case Action Subsystem5/2(In2)
  Merge1/1 -> state of B-dot mode (0/1)/1
  constant 1/1 -> Switch Case Action Subsystem7/2(Input1)
  Switch Case Action Subsystem5/1(Out1) -> Merge/1
  Switch Case Action Subsystem5/2(Out2) -> Merge1/1
  Switch Case Action Subsystem1/1(Out1) -> Merge/2
  Switch Case Action Subsystem1/2(Out2) -> Merge1/2
  Switch Case Action Subsystem2/1(Out1) -> Merge/3
  Switch Case Action Subsystem2/2(Out2) -> Merge1/3
  Switch Case Action Subsystem3/1(Out1) -> Merge/4
  Switch Case Action Subsystem3/2(Out2) -> Merge1/4
  Switch Case Action Subsystem4/1(Out1) -> Merge/5
  Switch Case Action Subsystem4/2(Out2) -> Merge1/5
  Switch Case Action Subsystem/1(Out1) -> Merge/7
  Switch Case Action Subsystem/2(Out2) -> Merge1/7
  Switch Case Action Subsystem7/1(Out1) -> Merge/6
  Switch Case Action Subsystem7/2(Out3) -> Merge1/6
  Switch Case/1 -> Switch Case Action Subsystem5/Action
  Switch Case/8 -> Switch Case Action Subsystem/Action
  Switch Case/7 -> Switch Case Action Subsystem6/Action
  Custom Quaternion_ECI/1 -> Switch Case Action Subsystem6/1(In1)
  Switch Case Action Subsystem6/1(Out1) -> Merge/8
  Switch Case Action Subsystem6/2(Out2) -> Merge1/8

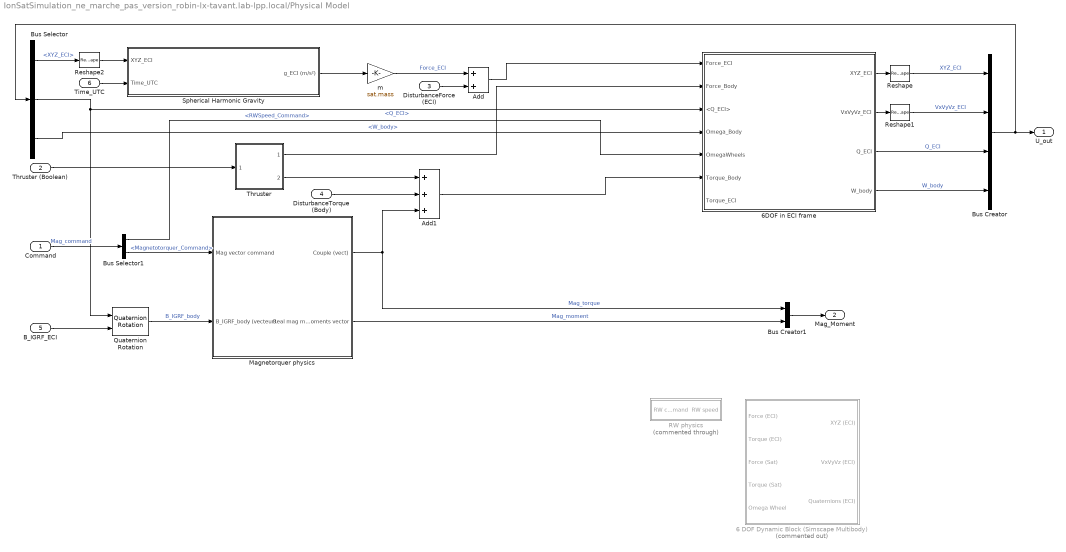
== system IonSatSimulation_ne_marche_pas_version_robin-lx-tavant.lab-lpp.local/Physical Model ==
  Command : Inport
  Thruster (Boolean) : Inport  Port=2
  DisturbanceForce (ECI) : Inport  Port=3
  DisturbanceTorque (Body) : Inport  Port=4
  B_IGRF_ECI : Inport  Port=5
  Time_UTC : Inport  Port=6
  6 DOF Dynamic Block (Simscape Multibody) : Subsystem  Commented=on
  6DOF in ECI frame : Subsystem
  Add : Sum
  Add1 : Sum  Inputs=+++
  Bus Creator : BusCreator  Inputs=4
  Bus Creator1 : BusCreator  Inputs=2
  Bus Selector : BusSelector  OutputSignals=XYZ_ECI,Q_ECI,W_body
  Bus Selector1 : BusSelector  OutputSignals=RWSpeed_Command,Magnetotorquer_Command
  Magnetorquer physics : Subsystem
  Quaternion Rotation : aerolibutil/Quaternion Rotation
  RW physics : Subsystem  Commented=through
  Reshape : Reshape
  Reshape1 : Reshape
  Reshape2 : Reshape  OutputDimensionality=Column vector (2-D)
  Spherical Harmonic Gravity : Subsystem  TreatAsAtomicUnit=on  SystemSampleTime=1
  Thruster : Subsystem
  m : Gain  Gain=sat.mass
  U_out : Outport
  Mag_Moment : Outport  Port=2
  wires:
  Bus Selector/1 -> Reshape2/1  "<XYZ_ECI>"
  Spherical Harmonic Gravity/1(g_ECI (m/s²)) -> m/1
  Thruster (Boolean)/1 -> Thruster/1(On/Off (Boolean))
  Bus Creator/1 -> Bus Selector/1, U_out/1
  Bus Selector/2 -> Quaternion Rotation/1, 6DOF in ECI frame/3(<Q_ECI>)  "<Q_ECI>"
  6DOF in ECI frame/3(Q_ECI) -> Bus Creator/3  "Q_ECI"
  6DOF in ECI frame/1(XYZ_ECI) -> Reshape/1
  6DOF in ECI frame/2(VxVyVz_ECI) -> Reshape1/1
  m/1 -> Add/1  "Force_ECI"
  Add/1 -> 6DOF in ECI frame/1(Force_ECI)
  Thruster/1(Force (G_sat)) -> 6DOF in ECI frame/2(Force_Body)
  Bus Selector1/2 -> Magnetorquer physics/1(Mag vector command)  "<Magnetotorquer_Command>"
  Thruster/2(Moment (G_sat)) -> Add1/1
  Add1/1 -> 6DOF in ECI frame/6(Torque_Body)
  DisturbanceForce (ECI)/1 -> Add/2
  DisturbanceTorque (Body)/1 -> Add1/2
  Reshape/1 -> Bus Creator/1  "XYZ_ECI"
  Reshape1/1 -> Bus Creator/2  "VxVyVz_ECI"
  Reshape2/1 -> Spherical Harmonic Gravity/1(XYZ_ECI)
  Bus Selector/3 -> 6DOF in ECI frame/4("Omega_Body ")  "<W_body>"
  Time_UTC/1 -> Spherical Harmonic Gravity/2(Time_UTC)
  B_IGRF_ECI/1 -> Quaternion Rotation/2
  Quaternion Rotation/1 -> Magnetorquer physics/2(B_IGRF_body (vecteur))  "B_IGRF_body"
  Magnetorquer physics/2(Real mag moments vector) -> Bus Creator1/2  "Mag_moment"
  Magnetorquer physics/1(Couple (vect)) -> Add1/3, Bus Creator1/1  "Mag_torque"
  6DOF in ECI frame/4(W_body) -> Bus Creator/4  "W_body"
  Command/1 -> Bus Selector1/1  "Mag_command"
  Bus Selector1/1 -> 6DOF in ECI frame/5(OmegaWheels)  "<RWSpeed_Command>"
  Bus Creator1/1 -> Mag_Moment/1

== system IonSatSimulation_ne_marche_pas_version_robin-lx-tavant.lab-lpp.local/QuatToAngleDeg ==
  In1 : Inport
  Abs : Abs
  Angle Conversion1 : aerolibconvert2/Angle Conversion  IU=rad  OU=deg
  Coordinate Transformation Conversion : robotcorelib/Coordinate Transformation Conversion  InputRepresentation=Quaternion  InputEulerSequence=ZYX  ShowTrVecInputPort=on  OutputRepresentation=Axis-Angle  OutputEulerSequence=ZYX  ShowTrVecOutputPort=on  SimulateUsing=Interpreted execution
      settings: SourceProductBaseCode=RO
  Demux1 : Demux
  Terminator1 : Terminator
  Terminator2 : Terminator
  Terminator3 : Terminator
  angle deg : Outport
  wires:
  In1/1 -> Coordinate Transformation Conversion/1
  Demux1/4 -> Angle Conversion1/1
  Demux1/1 -> Terminator1/1
  Coordinate Transformation Conversion/1 -> Demux1/1
  Angle Conversion1/1 -> Abs/1  "angle deg"
  Demux1/2 -> Terminator2/1
  Demux1/3 -> Terminator3/1
  Abs/1 -> angle deg/1

== system IonSatSimulation_ne_marche_pas_version_robin-lx-tavant.lab-lpp.local/Sensors ==
  B_ECI : Inport
  Sat-Sun vector : Inport  Port=2
  U : Inport  Port=3
  Bus Creator : BusCreator  Inputs=6
  MEMS Gyro : Subsystem
  Magnetometer : Subsystem
  Sun Sensor (Coarse) : Subsystem
  Sun Sensor (Sun sensor) : Subsystem
  Measurements : Outport
  wires:
  Sat-Sun vector/1 -> Sun Sensor (Coarse)/1(Sat-Sun_ECI), Sun Sensor (Sun sensor)/1(Sat-Sun_ECI)
  MEMS Gyro/1(W_Body_meas) -> Bus Creator/2  "W_body_meas"
  U/1 -> Magnetometer/1(U), MEMS Gyro/1(U), Sun Sensor (Coarse)/2(U), Sun Sensor (Sun sensor)/2(U)
  Magnetometer/1(B_Body_meas) -> Bus Creator/1  "B_Body_meas"
  Sun Sensor (Sun sensor)/1(Sat-Sun_precise_body_meas) -> Bus Creator/3  "Sun_precise_Body_meas"
  Sun Sensor (Coarse)/1(Sat-Sun_coarse_body_meas) -> Bus Creator/5  "Sun_coarse_Body_meas"
  Sun Sensor (Sun sensor)/2(Sensor active (bool)) -> Bus Creator/4  "ActiveCubesense"
  Sun Sensor (Coarse)/2(Sensor active (bool)) -> Bus Creator/6  "ActiveCoarse"
  Bus Creator/1 -> Measurements/1
  B_ECI/1 -> Magnetometer/2(B_IGRF_ECI)

== system IonSatSimulation_ne_marche_pas_version_robin-lx-tavant.lab-lpp.local/Signal Logging ==
  U : Inport
  Command : Inport  Port=2
  Qc : Inport  Port=3
  Bus Selector : BusSelector  OutputSignals=RWSpeed_Command,Magnetotorquer_Command
  Bus Selector4 : BusSelector  OutputSignals=XYZ_ECI,VxVyVz_ECI,Q_ECI,W_body
  Reshape : Reshape
  Reshape1 : Reshape
  Reshape2 : Reshape
  To Workspace : ToWorkspace  VariableName=sat_pos  SaveFormat=Timeseries  SampleTime=1
      settings: Save2DSignal=2-D array (concatenate along first dimension)
  To Workspace1 : ToWorkspace  VariableName=sat_speed  SaveFormat=Timeseries  SampleTime=1
      settings: Save2DSignal=2-D array (concatenate along first dimension)
  To Workspace2 : ToWorkspace  VariableName=sat_Q  SaveFormat=Timeseries  SampleTime=1
      settings: Save2DSignal=2-D array (concatenate along first dimension)
  To Workspace3 : ToWorkspace  VariableName=sat_omega  SaveFormat=Timeseries  SampleTime=1
      settings: Save2DSignal=2-D array (concatenate along first dimension)
  To Workspace4 : ToWorkspace  VariableName=RWSpeed_Command  SaveFormat=Timeseries  SampleTime=1
      settings: Save2DSignal=2-D array (concatenate along first dimension)
  To Workspace5 : ToWorkspace  VariableName=sat_Qc  SaveFormat=Timeseries  SampleTime=1
      settings: Save2DSignal=2-D array (concatenate along first dimension)
  To Workspace6 : ToWorkspace  VariableName=Mag_Command  SaveFormat=Timeseries  SampleTime=1
      settings: Save2DSignal=2-D array (concatenate along first dimension)
  wires:
  Bus Selector4/3 -> To Workspace2/1  "<Q_ECI>"
  Bus Selector4/4 -> To Workspace3/1  "<W_body>"
  U/1 -> Bus Selector4/1
  Bus Selector4/2 -> To Workspace1/1  "<VxVyVz_ECI>"
  Command/1 -> Bus Selector/1
  Bus Selector4/1 -> To Workspace/1  "<XYZ_ECI>"
  Qc/1 -> Reshape1/1
  Reshape/1 -> To Workspace4/1
  Reshape1/1 -> To Workspace5/1
  Bus Selector/1 -> Reshape/1  "<RWSpeed_Command>"
  Bus Selector/2 -> Reshape2/1  "<Magnetotorquer_Command>"
  Reshape2/1 -> To Workspace6/1

== system IonSatSimulation_ne_marche_pas_version_robin-lx-tavant.lab-lpp.local/Time propagator ==
  Add : Sum  Inputs=|++
  Clock : Clock
  Constant : Constant  Value=86400
  Day : Constant
  Divide : Product  Inputs=*/
  HH : Constant  Value=0
  JD to UTC : MATLAB Function  TreatAsAtomicUnit=on
  MM : Constant  Value=0
  Month : Constant
  Mux : Mux  Inputs=6
  Reshape : Reshape
  SS : Constant  Value=0
  Signal logging : ToWorkspace  VariableName=T_UTC  SaveFormat=Timeseries  SampleTime=1
      settings: Save2DSignal=2-D array (concatenate along first dimension)
  Signal logging1 : ToWorkspace  VariableName=T_JD  SaveFormat=Timeseries  SampleTime=1
      settings: Save2DSignal=2-D array (concatenate along first dimension)
  UTC to JD : MATLAB Function  TreatAsAtomicUnit=on
  Year : Constant  Value=2022
  T_UTC : Outport
  T_JD : Outport  Port=2
  wires:
  UTC to JD/1(JD) -> Add/1  "JD_0"
  Clock/1 -> Divide/1
  Constant/1 -> Divide/2
  JD to UTC/1(Time_UTC) -> T_UTC/1, Reshape/1
  Divide/1 -> Add/2
  Mux/1 -> UTC to JD/1(Time_UTC)
  Day/1 -> Mux/3
  Month/1 -> Mux/2
  Year/1 -> Mux/1
  HH/1 -> Mux/4
  MM/1 -> Mux/5
  SS/1 -> Mux/6
  Reshape/1 -> Signal logging/1
  Add/1 -> Signal logging1/1, T_JD/1, JD to UTC/1(JD)

== system IonSatSimulation_ne_marche_pas_version_robin-lx-tavant.lab-lpp.local/Basic Gravity (first order)/Norm ==
  u : Inport
  Abs : Abs
  Add : Sum  Inputs=+++
  Demux1 : Demux  Outputs=3
  Square : Math  Operator=square  SaturateOnIntegerOverflow=on
  Square1 : Math  Operator=square  SaturateOnIntegerOverflow=on
  Square2 : Math  Operator=square  SaturateOnIntegerOverflow=on
  r**2 : Outport
  wires:
  Demux1/2 -> Square1/1
  Add/1 -> r**2/1  "r**2"
  Square/1 -> Add/1
  u/1 -> Abs/1
  Demux1/1 -> Square/1
  Demux1/3 -> Square2/1
  Abs/1 -> Demux1/1
  Square2/1 -> Add/3
  Square1/1 -> Add/2

== system IonSatSimulation_ne_marche_pas_version_robin-lx-tavant.lab-lpp.local/Controller/B-dot choice1 ==
  " command (normal)" : Inport
  Command (B-dot) : Inport  Port=2
  B_dot mode (0/1) : Inport  Port=3
  If1 : If
  Merge : Merge
  Switch Case Action Subsystem3 : Subsystem  TreatAsAtomicUnit=on
  Switch Case Action Subsystem4 : Subsystem  TreatAsAtomicUnit=on
  output command : Outport
  wires:
  " command (normal)"/1 -> Switch Case Action Subsystem4/1(In1)
  If1/2 -> Switch Case Action Subsystem4/Action
  If1/1 -> Switch Case Action Subsystem3/Action
  B_dot mode (0/1)/1 -> If1/1
  Command (B-dot)/1 -> Switch Case Action Subsystem3/1(In1)
  Merge/1 -> output command/1
  Switch Case Action Subsystem3/1(Out1) -> Merge/1
  Switch Case Action Subsystem4/1(Out1) -> Merge/2

== system IonSatSimulation_ne_marche_pas_version_robin-lx-tavant.lab-lpp.local/Controller/B-dot choice2 ==
  " command (normal)" : Inport
  Command (B-dot) : Inport  Port=2
  B_dot mode (0/1) : Inport  Port=3
  If1 : If
  Merge : Merge
  Switch Case Action Subsystem3 : Subsystem  TreatAsAtomicUnit=on
  Switch Case Action Subsystem4 : Subsystem  TreatAsAtomicUnit=on
  output command : Outport
  wires:
  " command (normal)"/1 -> Switch Case Action Subsystem4/1(In1)
  If1/2 -> Switch Case Action Subsystem4/Action
  If1/1 -> Switch Case Action Subsystem3/Action
  B_dot mode (0/1)/1 -> If1/1
  Command (B-dot)/1 -> Switch Case Action Subsystem3/1(In1)
  Merge/1 -> output command/1
  Switch Case Action Subsystem3/1(Out1) -> Merge/1
  Switch Case Action Subsystem4/1(Out1) -> Merge/2

== system IonSatSimulation_ne_marche_pas_version_robin-lx-tavant.lab-lpp.local/Controller/B-dot command ==
  note: ref : OneDrive\IonSat X18\SCAO\Contrôle attitude\Detumbling\Detumbling and Aerostable Control for Cubesats.pdf
      |
      | formulae:
      | $\mathbf{\dot B} \simeq \mathbf{B}\times \mathbf{\dot \theta}$
      | $\mathbf{m} = -c\mathbf{\dot B}$
      |
      | this block does NOT decide if the B-dot mode is relevant or not
      | (it applies it without question on the rotation rate :
      | $\Omega=v/r= \sqrt{\frac{Gm_{earth}}{(h+r_{earth})^{3/2}}} \sim 0.066 °/s$ So the command MUST stop the B-dot mode when the estimated rotation speed is smaller than 0.1 degree per second )
  note: entrée:
      | champ magnétique
      | sortie: moment magnetique de commande et vitesse des roues à réaction (nulle)
  B : Inport
  Discrete Derivative : simulink/Discrete/Discrete Derivative  gainval=1.0  ICPrevScaledInput=0.0  OutMin=[]  OutMax=[]  OutDataType=fixdt(1, 16)  OutScaling=2^-10  DoSatur=off
  Divide1 : Product  Inputs=**
  Reshape2 : Reshape  OutputDimensionality=Column vector (2-D)
  constant c : Constant  Value=-sat.bdot_c
  wheels unused : Constant  Value=[0, 0, 0]
  Magnetic moment (B-dot) : Outport
  Wheel command (0) : Outport  Port=2
  wires:
  constant c/1 -> Divide1/2
  B/1 -> Discrete Derivative/1
  Discrete Derivative/1 -> Divide1/1  "B_point=B^theta_point"
  Divide1/1 -> Magnetic moment (B-dot)/1
  wheels unused/1 -> Reshape2/1
  Reshape2/1 -> Wheel command (0)/1

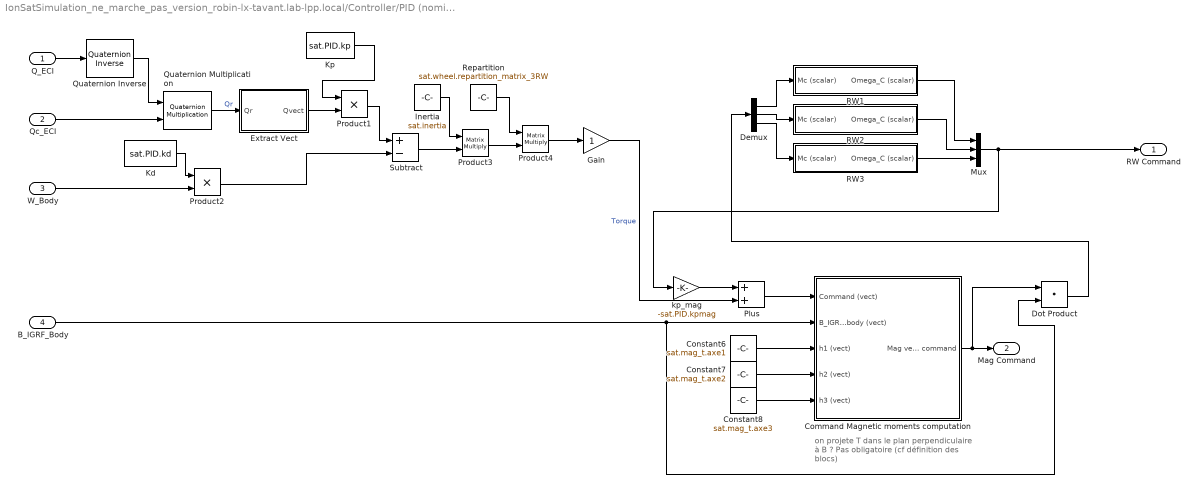
== system IonSatSimulation_ne_marche_pas_version_robin-lx-tavant.lab-lpp.local/Controller/PID (nominal command) ==
  note: on projete T dans
      | le plan perpendiculaire à B ?
      | Pas obligatoire (cf définition des blocs)
  Q_ECI : Inport
  Qc_ECI : Inport  Port=2
  W_Body : Inport  Port=3
  B_IGRF_Body : Inport  Port=4
  Command Magnetic moments computation : Subsystem
  Constant6 : Constant  Value=sat.mag_t.axe1
  Constant7 : Constant  Value=sat.mag_t.axe2
  Constant8 : Constant  Value=sat.mag_t.axe3
  Demux : Demux  Outputs=3
  Dot Product : DotProduct  InputSameDT=on  OutDataTypeStr=Inherit: Inherit via internal rule
  Extract Vect : Subsystem
  Gain : Gain
  Inertia : Constant  Value=sat.inertia
  Kd : Constant  Value=sat.PID.kd
  Kp : Constant  Value=sat.PID.kp
  Mux : Mux  Inputs=3
  Plus : Sum
  Product1 : Product
  Product2 : Product
  Product3 : Product  Multiplication=Matrix(*)
  Product4 : Product  Multiplication=Matrix(*)
  Quaternion Inverse : aerolibutil/Quaternion Inverse
      settings: SourceProductName=Aerospace Blockset
  Quaternion Multiplication : aerolibutil/Quaternion Multiplication
  RW1 : Subsystem
  RW2 : Subsystem
  RW3 : Subsystem
  Repartition : Constant  Value=sat.wheel.repartition_matrix_3RW
  Subtract : Sum  Inputs=+-
  kp_mag : Gain  Gain=-sat.PID.kpmag
  RW Command : Outport
  Mag Command : Outport  Port=2
  wires:
  RW1/1(Omega_C (scalar)) -> Mux/1
  Q_ECI/1 -> Quaternion Inverse/1
  Demux/3 -> RW3/1(Mc (scalar))
  Constant7/1 -> Command Magnetic moments computation/4(h2 (vect))
  Extract Vect/1(Qvect) -> Product1/2
  Mux/1 -> kp_mag/1, RW Command/1
  Demux/1 -> RW1/1(Mc (scalar))
  Kd/1 -> Product2/1
  Constant6/1 -> Command Magnetic moments computation/3(h1 (vect))
  Constant8/1 -> Command Magnetic moments computation/5(h3 (vect))
  Command Magnetic moments computation/1(Mag vector command) -> Dot Product/1, Mag Command/1
  Product4/1 -> Gain/1
  RW3/1(Omega_C (scalar)) -> Mux/3
  Kp/1 -> Product1/1
  Repartition/1 -> Product4/1
  RW2/1(Omega_C (scalar)) -> Mux/2
  Demux/2 -> RW2/1(Mc (scalar))
  Product1/1 -> Subtract/1
  Subtract/1 -> Product3/2
  Quaternion Inverse/1 -> Quaternion Multiplication/1
  Inertia/1 -> Product3/1
  Quaternion Multiplication/1 -> Extract Vect/1(Qr)  "Qr"
  Product3/1 -> Product4/2
  Product2/1 -> Subtract/2
  W_Body/1 -> Product2/2
  Qc_ECI/1 -> Quaternion Multiplication/2
  B_IGRF_Body/1 -> Dot Product/2, Command Magnetic moments computation/2(B_IGRF_body (vect))
  kp_mag/1 -> Plus/1
  Plus/1 -> Command Magnetic moments computation/1(Command (vect))
  Gain/1 -> Plus/2  "Torque"
  Dot Product/1 -> Demux/1

== system IonSatSimulation_ne_marche_pas_version_robin-lx-tavant.lab-lpp.local/Controller/RW4 ==
  note: Entrées:
      | - Moment de commande (déjà projeté sur l'axe de la roue...)
      | Sorties:
      | - Omega de commande à appliquer
  Mc (scalar) : Inport
  Divide : Product  Inputs=*/
  Saturation_speed : Saturate  UpperLimit=sat.wheel.max_speed  LowerLimit=- sat.wheel.max_speed
  Torque_sat : Saturate  UpperLimit=sat.wheel.max_torque  LowerLimit=- sat.wheel.max_torque
  Wheel Inertia : Constant  Value=sat.wheel.max_sigma/sat.wheel.max_speed
  Omega_C (scalar) : Outport  VectorParamsAs1DForOutWhenUnconnected=on
  wires:
  Mc (scalar)/1 -> Torque_sat/1
  Wheel Inertia/1 -> Divide/2
  Divide/1 -> ?  "dw/dt"
  ? -> Saturation_speed/1
  Torque_sat/1 -> Divide/1  "Torque (scal)"
  Saturation_speed/1 -> Omega_C (scalar)/1

== system IonSatSimulation_ne_marche_pas_version_robin-lx-tavant.lab-lpp.local/Kalmann Filter/Coarse Sun Sensor ==
  Sat-Sun_ECI : Inport
  SunMeasure : TriggerPort  TriggerType=function-call  IsSimulinkFunction=on  FunctionName=SunMeasureCoarse  FunctionVisibility=scoped  VariantControl=(inherit)
  Demux : Demux  Outputs=2
  Quaternion Rotation1 : aerolibutil/Quaternion Rotation
  Terminator : Terminator
  u : ArgIn  DisableCoverage=on  PortDimensions=7  ArgumentName=u
  y : ArgOut  DisableCoverage=on  PortDimensions=3  ArgumentName=y
  wires:
  Quaternion Rotation1/1 -> y/1  "Sat_Sun_body"
  Sat-Sun_ECI/1 -> Quaternion Rotation1/2
  Demux/2 -> Terminator/1
  Demux/1 -> Quaternion Rotation1/1
  u/1 -> Demux/1
